simulink model "hbtc_ut"  (Simulink 8.1)
settings: Solver=FixedStepDiscrete  StartTime=0.0  StopTime=Inf  FixedStep=0.005  RelTol=1e-3
libraries: siltestlib x3, hbtc x1
settings Model: Creator=xsellart  LastModifiedBy=AT015555
settings DataIOCC: SignalLoggingSaveFormat=Dataset
settings OptimizationCC: ExpressionDepthLimit=128
settings DebuggingCC: FcnCallInpInsideContextMsg=EnableAllAsError
settings GRTTargetCC: CombineOutputUpdateFcns=on  GRTInterface=off

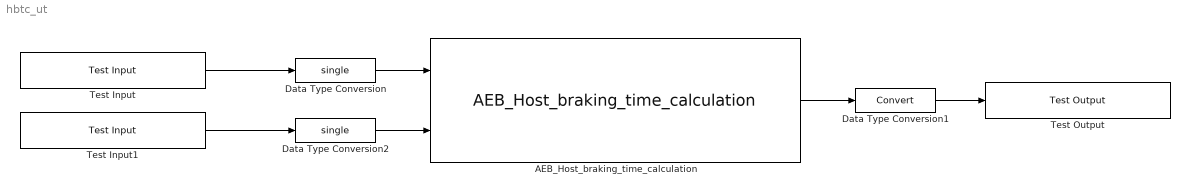
== system hbtc_ut ==
  AEB_Host_braking_time_calculation : hbtc/AEB_Host_braking_time_calculation
  Data Type Conversion : DataTypeConversion  OutDataTypeStr=single
  Data Type Conversion1 : DataTypeConversion
  Data Type Conversion2 : DataTypeConversion  OutDataTypeStr=single
  Test Input : siltestlib/Test Input  varname=VDINR_VehSpd_mps  sampletime=0.005
  Test Input1 : siltestlib/Test Input  varname=VJUD_ConsideredDecel_mps2  sampletime=0.005
  Test Output : siltestlib/Test Output  varname=VJUD_HostBrakingTime_sec  sampletime=-1
  wires:
  Data Type Conversion1/1 -> Test Output/1
  Test Input/1 -> Data Type Conversion/1
  Data Type Conversion/1 -> AEB_Host_braking_time_calculation/1
  AEB_Host_braking_time_calculation/1 -> Data Type Conversion1/1
  Test Input1/1 -> Data Type Conversion2/1
  Data Type Conversion2/1 -> AEB_Host_braking_time_calculation/2
